simulink model "AccelCtrl_ACC"  (Simulink 7.5)
settings: Solver=ode45  StartTime=0.0  StopTime=inf  RelTol=1e-3
libraries: CarMaker4SL x31, simulink x2
(part 2 of 2)

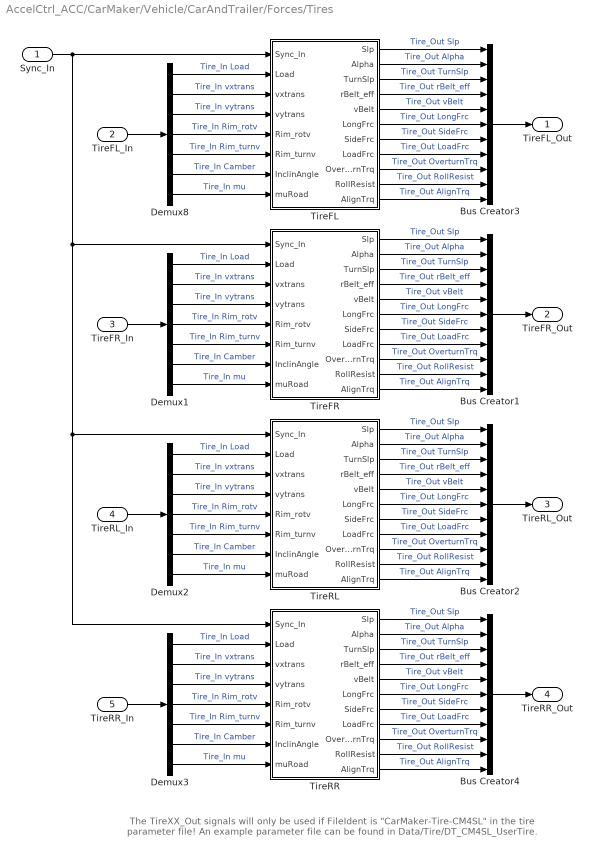
== system AccelCtrl_ACC/CarMaker/Vehicle/CarAndTrailer/Forces/Tires ==
  note: The TireXX_Out signals will only be used if FileIdent is "CarMaker-Tire-CM4SL" in the tire parameter file!
      | An example parameter file can be found in Data/Tire/DT_CM4SL_UserTire.
  Sync_In : Inport  OutDataType=sfix(16)  OutScaling=2^0
  TireFL_In : Inport  Port=2  OutDataType=sfix(16)  OutScaling=2^0
  TireFR_In : Inport  Port=3  OutDataType=sfix(16)  OutScaling=2^0
  TireRL_In : Inport  Port=4  OutDataType=sfix(16)  OutScaling=2^0
  TireRR_In : Inport  Port=5  OutDataType=sfix(16)  OutScaling=2^0
  Bus Creator{1..4} (4 alike) : BusCreator  Inputs=11
  Demux{1..3,8} (4 alike) : Demux  Outputs=7
  TireFL : Subsystem
  TireFR : Subsystem
  TireRL : Subsystem
  TireRR : Subsystem
  TireFL_Out : Outport  OutDataType=sfix(16)  OutScaling=2^0
  TireFR_Out : Outport  Port=2  OutDataType=sfix(16)  OutScaling=2^0
  TireRL_Out : Outport  Port=3  OutDataType=sfix(16)  OutScaling=2^0
  TireRR_Out : Outport  Port=4  OutDataType=sfix(16)  OutScaling=2^0
  wires:
  Sync_In/1 -> TireRR/1(Sync_In), TireRL/1(Sync_In), TireFR/1(Sync_In), TireFL/1(Sync_In)
  Bus Creator4/1 -> TireRR_Out/1
  Bus Creator2/1 -> TireRL_Out/1
  Bus Creator1/1 -> TireFR_Out/1
  Demux3/5 -> TireRR/6(Rim_turnv)  "Tire_In Rim_turnv"
  Demux3/4 -> TireRR/5(Rim_rotv)  "Tire_In Rim_rotv"
  Demux3/1 -> TireRR/2(Load)  "Tire_In Load"
  Demux3/7 -> TireRR/8(muRoad)  "Tire_In mu"
  Demux3/6 -> TireRR/7(InclinAngle)  "Tire_In Camber"
  Demux3/2 -> TireRR/3(vxtrans)  "Tire_In vxtrans"
  Demux3/3 -> TireRR/4(vytrans)  "Tire_In vytrans"
  TireRR/11(AlignTrq) -> Bus Creator4/11  "Tire_Out AlignTrq"
  TireRR/10(RollResist) -> Bus Creator4/10  "Tire_Out RollResist"
  TireRR/9(OverturnTrq) -> Bus Creator4/9  "Tire_Out OverturnTrq"
  TireRR/8(LoadFrc) -> Bus Creator4/8  "Tire_Out LoadFrc"
  TireRR/7(SideFrc) -> Bus Creator4/7  "Tire_Out SideFrc"
  TireRR/6(LongFrc) -> Bus Creator4/6  "Tire_Out LongFrc"
  TireRR/5(vBelt) -> Bus Creator4/5  "Tire_Out vBelt"
  TireRR/4(rBelt_eff) -> Bus Creator4/4  "Tire_Out rBelt_eff"
  TireRR/3(TurnSlp) -> Bus Creator4/3  "Tire_Out TurnSlp"
  TireRR/1(Slp) -> Bus Creator4/1  "Tire_Out Slp"
  TireRR/2(Alpha) -> Bus Creator4/2  "Tire_Out Alpha"
  Demux2/5 -> TireRL/6(Rim_turnv)  "Tire_In Rim_turnv"
  Demux2/4 -> TireRL/5(Rim_rotv)  "Tire_In Rim_rotv"
  Demux2/1 -> TireRL/2(Load)  "Tire_In Load"
  Demux2/7 -> TireRL/8(muRoad)  "Tire_In mu"
  Demux2/6 -> TireRL/7(InclinAngle)  "Tire_In Camber"
  Demux2/2 -> TireRL/3(vxtrans)  "Tire_In vxtrans"
  Demux2/3 -> TireRL/4(vytrans)  "Tire_In vytrans"
  TireRL/11(AlignTrq) -> Bus Creator2/11  "Tire_Out AlignTrq"
  TireRL/10(RollResist) -> Bus Creator2/10  "Tire_Out RollResist"
  TireRL/9(OverturnTrq) -> Bus Creator2/9  "Tire_Out OverturnTrq"
  TireRL/8(LoadFrc) -> Bus Creator2/8  "Tire_Out LoadFrc"
  TireRL/7(SideFrc) -> Bus Creator2/7  "Tire_Out SideFrc"
  TireRL/6(LongFrc) -> Bus Creator2/6  "Tire_Out LongFrc"
  TireRL/5(vBelt) -> Bus Creator2/5  "Tire_Out vBelt"
  TireRL/4(rBelt_eff) -> Bus Creator2/4  "Tire_Out rBelt_eff"
  TireRL/3(TurnSlp) -> Bus Creator2/3  "Tire_Out TurnSlp"
  TireRL/1(Slp) -> Bus Creator2/1  "Tire_Out Slp"
  TireRL/2(Alpha) -> Bus Creator2/2  "Tire_Out Alpha"
  Demux1/5 -> TireFR/6(Rim_turnv)  "Tire_In Rim_turnv"
  Demux1/4 -> TireFR/5(Rim_rotv)  "Tire_In Rim_rotv"
  Demux1/1 -> TireFR/2(Load)  "Tire_In Load"
  Demux1/7 -> TireFR/8(muRoad)  "Tire_In mu"
  Demux1/6 -> TireFR/7(InclinAngle)  "Tire_In Camber"
  Demux1/2 -> TireFR/3(vxtrans)  "Tire_In vxtrans"
  Demux1/3 -> TireFR/4(vytrans)  "Tire_In vytrans"
  TireFR/11(AlignTrq) -> Bus Creator1/11  "Tire_Out AlignTrq"
  TireFR/10(RollResist) -> Bus Creator1/10  "Tire_Out RollResist"
  TireFR/9(OverturnTrq) -> Bus Creator1/9  "Tire_Out OverturnTrq"
  TireFR/8(LoadFrc) -> Bus Creator1/8  "Tire_Out LoadFrc"
  TireFR/7(SideFrc) -> Bus Creator1/7  "Tire_Out SideFrc"
  TireFR/6(LongFrc) -> Bus Creator1/6  "Tire_Out LongFrc"
  TireFR/5(vBelt) -> Bus Creator1/5  "Tire_Out vBelt"
  TireFR/4(rBelt_eff) -> Bus Creator1/4  "Tire_Out rBelt_eff"
  TireFR/3(TurnSlp) -> Bus Creator1/3  "Tire_Out TurnSlp"
  TireFR/1(Slp) -> Bus Creator1/1  "Tire_Out Slp"
  TireFR/2(Alpha) -> Bus Creator1/2  "Tire_Out Alpha"
  Demux8/5 -> TireFL/6(Rim_turnv)  "Tire_In Rim_turnv"
  Demux8/4 -> TireFL/5(Rim_rotv)  "Tire_In Rim_rotv"
  TireFL_In/1 -> Demux8/1
  Demux8/1 -> TireFL/2(Load)  "Tire_In Load"
  Demux8/7 -> TireFL/8(muRoad)  "Tire_In mu"
  Demux8/6 -> TireFL/7(InclinAngle)  "Tire_In Camber"
  Demux8/2 -> TireFL/3(vxtrans)  "Tire_In vxtrans"
  Demux8/3 -> TireFL/4(vytrans)  "Tire_In vytrans"
  TireFL/11(AlignTrq) -> Bus Creator3/11  "Tire_Out AlignTrq"
  TireFL/10(RollResist) -> Bus Creator3/10  "Tire_Out RollResist"
  TireFL/9(OverturnTrq) -> Bus Creator3/9  "Tire_Out OverturnTrq"
  TireFL/8(LoadFrc) -> Bus Creator3/8  "Tire_Out LoadFrc"
  TireFL/7(SideFrc) -> Bus Creator3/7  "Tire_Out SideFrc"
  TireFL/6(LongFrc) -> Bus Creator3/6  "Tire_Out LongFrc"
  TireFL/5(vBelt) -> Bus Creator3/5  "Tire_Out vBelt"
  TireFL/4(rBelt_eff) -> Bus Creator3/4  "Tire_Out rBelt_eff"
  TireFL/3(TurnSlp) -> Bus Creator3/3  "Tire_Out TurnSlp"
  TireFL/1(Slp) -> Bus Creator3/1  "Tire_Out Slp"
  TireFL/2(Alpha) -> Bus Creator3/2  "Tire_Out Alpha"
  Bus Creator3/1 -> TireFL_Out/1
  TireFR_In/1 -> Demux1/1
  TireRL_In/1 -> Demux2/1
  TireRR_In/1 -> Demux3/1

== system AccelCtrl_ACC/CarMaker/Vehicle/CarAndTrailer/Forces/Vehicle Forces ==
  Sync_In : Inport  OutDataType=sfix(16)  OutScaling=2^0
  Bus Creator1 : BusCreator  Inputs=12
  Bus Creator5 : BusCreator  Inputs=13
  Bus Creator8 : BusCreator  Inputs=16
  Demux : Demux  Outputs=16
  Demux1 : Demux  Outputs=12
  Demux5 : Demux  Outputs=13
  Forces : S-Function  FunctionName=CM_Sfun  Parameters='Forces'  EnableBusSupport=off
  Sync_Out : Outport  OutDataType=sfix(16)  OutScaling=2^0
  Car.Virtual : Outport  Port=2  OutDataType=sfix(16)  OutScaling=2^0
  Car.Aero : Outport  Port=3  OutDataType=sfix(16)  OutScaling=2^0
  Car.Load : Outport  Port=4  OutDataType=sfix(16)  OutScaling=2^0
  wires:
  Demux5/7 -> Bus Creator5/7  "car Aero vRes_1 z"
  Demux5/6 -> Bus Creator5/6  "car Aero vRes_1 y"
  Demux5/5 -> Bus Creator5/5  "car Aero vRes_1 x"
  Demux5/4 -> Bus Creator5/4  "Vehicle Wind_vel_0 z"
  Demux5/3 -> Bus Creator5/3  "Vehicle Wind_vel_0 y"
  Demux5/2 -> Bus Creator5/2  "Vehicle Wind_vel_0 x"
  Demux5/1 -> Bus Creator5/1  "Vehicle sRoadAero"
  Demux5/8 -> Bus Creator5/8  "car Aero Frc_1 x"
  Demux5/9 -> Bus Creator5/9  "car Aero Frc_1 y"
  Demux5/10 -> Bus Creator5/10  "car Aero Frc_1 z"
  Demux5/13 -> Bus Creator5/13  "car Aero Trq_1 z"
  Demux5/12 -> Bus Creator5/12  "car Aero Trq_1 y"
  Demux5/11 -> Bus Creator5/11  "car Aero Trq_1 x"
  Forces/4 -> Demux/1
  Demux/12 -> Bus Creator8/12  "Car Load_2 tz"
  Demux/11 -> Bus Creator8/11  "Car Load_2 ty"
  Demux/10 -> Bus Creator8/10  "Car Load_2 tx"
  Demux/9 -> Bus Creator8/9  "Car Load_2 mass"
  Demux/8 -> Bus Creator8/8  "Car Load_1 tz"
  Demux/7 -> Bus Creator8/7  "Car Load_1 ty"
  Demux/6 -> Bus Creator8/6  "Car Load_1 tx"
  Demux/5 -> Bus Creator8/5  "Car Load_1 mass"
  Demux/4 -> Bus Creator8/4  "Car Load_0 tz"
  Demux/3 -> Bus Creator8/3  "Car Load_0 ty"
  Demux/2 -> Bus Creator8/2  "Car Load_0 tx"
  Demux/1 -> Bus Creator8/1  "Car Load_0 mass"
  Bus Creator8/1 -> Car.Load/1
  Bus Creator1/1 -> Car.Virtual/1
  Forces/2 -> Demux1/1
  Forces/3 -> Demux5/1
  Demux1/3 -> Bus Creator1/3  "Car Virtual Frc_1 z"
  Demux1/2 -> Bus Creator1/2  "Car Virtual Frc_1 y"
  Demux1/1 -> Bus Creator1/1  "Car Virtual Frc_1 x"
  Bus Creator5/1 -> Car.Aero/1
  Forces/1 -> Sync_Out/1
  Sync_In/1 -> Forces/1
  Demux1/4 -> Bus Creator1/4  "Car Virtual Frc_0 x"
  Demux1/5 -> Bus Creator1/5  "Car Virtual Frc_0 y"
  Demux1/6 -> Bus Creator1/6  "Car Virtual Frc_0 z"
  Demux1/7 -> Bus Creator1/7  "Car Virtual Trq_1 x"
  Demux1/8 -> Bus Creator1/8  "Car Virtual Trq_1 y"
  Demux1/9 -> Bus Creator1/9  "Car Virtual Trq_1 z"
  Demux1/10 -> Bus Creator1/10  "Car Virtual Trq_0 x"
  Demux1/11 -> Bus Creator1/11  "Car Virtual Trq_0 y"
  Demux1/12 -> Bus Creator1/12  "Car Virtual Trq_0 z"
  Demux/13 -> Bus Creator8/13  "Car Load_3 mass"
  Demux/14 -> Bus Creator8/14  "Car Load_3 tx"
  Demux/15 -> Bus Creator8/15  "Car Load_3 ty"
  Demux/16 -> Bus Creator8/16  "Car Load_3 tz"

== system AccelCtrl_ACC/CarMaker/Vehicle/CarAndTrailer/Trailer/CreateBus Car.Hitch.FrcTrq ==
  In1 : Inport  OutDataType=sfix(16)  OutScaling=2^0
  Bus Creator7 : BusCreator  Inputs=6
  Demux7 : Demux  Outputs=6
  Car.Hitch.FrcTrq : Outport  OutDataType=sfix(16)  OutScaling=2^0
  wires:
  Demux7/1 -> Bus Creator7/1  "Car Hitch Frc2Car x"
  Demux7/2 -> Bus Creator7/2  "Car Hitch Frc2Car y"
  Demux7/3 -> Bus Creator7/3  "Car Hitch Frc2Car z"
  Demux7/4 -> Bus Creator7/4  "Car Hitch Trq2Car x"
  Demux7/5 -> Bus Creator7/5  "Car Hitch Trq2Car y"
  Demux7/6 -> Bus Creator7/6  "Car Hitch Trq2Car z"
  Bus Creator7/1 -> Car.Hitch.FrcTrq/1
  In1/1 -> Demux7/1

== system AccelCtrl_ACC/CarMaker/Vehicle/CarAndTrailer/Trailer/CreateBus Vhcl.Motion ==
  In1 : Inport  OutDataType=sfix(16)  OutScaling=2^0
  Demux1 : Demux  Outputs=16
  Mux1 : Mux  Inputs=16
  Out1 : Outport  OutDataType=sfix(16)  OutScaling=2^0
  wires:
  Mux1/1 -> Out1/1
  In1/1 -> Demux1/1
  Demux1/16 -> Mux1/16  "Vhcl YawAcc"
  Demux1/15 -> Mux1/15  "Vhcl YawRate"
  Demux1/14 -> Mux1/14  "Vhcl Yaw"
  Demux1/13 -> Mux1/13  "Vhcl PitchAcc"
  Demux1/12 -> Mux1/12  "Vhcl PitchVel"
  Demux1/11 -> Mux1/11  "Vhcl Pitch"
  Demux1/10 -> Mux1/10  "Vhcl RollAcc"
  Demux1/9 -> Mux1/9  "Vhcl RollVel"
  Demux1/8 -> Mux1/8  "Vhcl Roll"
  Demux1/7 -> Mux1/7  "Vhcl Hitch_Pos z"
  Demux1/6 -> Mux1/6  "Vhcl Hitch_Pos y"
  Demux1/5 -> Mux1/5  "Vhcl Hitch_Pos x"
  Demux1/4 -> Mux1/4  "Vhcl sRoadAero"
  Demux1/3 -> Mux1/3  "Vhcl sRoad"
  Demux1/2 -> Mux1/2  "Vhcl Distance"
  Demux1/1 -> Mux1/1  "Vhcl v"

== system AccelCtrl_ACC/CarMaker/Vehicle/CarAndTrailer/Trailer/CreateBus Vhcl.PoI ==
  In1 : Inport  OutDataType=sfix(16)  OutScaling=2^0
  Bus Creator3 : BusCreator  Inputs=18
  Demux3 : Demux  Outputs=18
  Out1 : Outport  OutDataType=sfix(16)  OutScaling=2^0
  wires:
  Demux3/1 -> Bus Creator3/1  "Vhcl PoI_Pos x"
  Bus Creator3/1 -> Out1/1
  In1/1 -> Demux3/1
  Demux3/2 -> Bus Creator3/2  "Vhcl PoI_Pos y"
  Demux3/3 -> Bus Creator3/3  "Vhcl PoI_Pos z"
  Demux3/4 -> Bus Creator3/4  "Vhcl PoI_Vel x"
  Demux3/5 -> Bus Creator3/5  "Vhcl PoI_Vel y"
  Demux3/6 -> Bus Creator3/6  "Vhcl PoI_Vel z"
  Demux3/7 -> Bus Creator3/7  "Vhcl PoI_Acc x"
  Demux3/8 -> Bus Creator3/8  "Vhcl PoI_Acc y"
  Demux3/9 -> Bus Creator3/9  "Vhcl PoI_Acc z"
  Demux3/10 -> Bus Creator3/10  "Vhcl PoI_Vel_1 x"
  Demux3/11 -> Bus Creator3/11  "Vhcl PoI_Vel_1 y"
  Demux3/12 -> Bus Creator3/12  "Vhcl PoI_Vel_1 z"
  Demux3/13 -> Bus Creator3/13  "Vhcl PoI_Acc_1 x"
  Demux3/14 -> Bus Creator3/14  "Vhcl PoI_Acc_1 y"
  Demux3/15 -> Bus Creator3/15  "Vhcl PoI_Acc_1 z"
  Demux3/16 -> Bus Creator3/16  "Vhcl PoI_GCS Long"
  Demux3/17 -> Bus Creator3/17  "Vhcl PoI_GCS Lat"
  Demux3/18 -> Bus Creator3/18  "Vhcl PoI_GCS Elev"

== system AccelCtrl_ACC/CarMaker/Vehicle/CarAndTrailer/Trailer/CreateBus Vhcl.Steering ==
  In1 : Inport  OutDataType=sfix(16)  OutScaling=2^0
  Bus Creator3 : BusCreator
  Demux : Demux
  Out1 : Outport  OutDataType=sfix(16)  OutScaling=2^0
  wires:
  In1/1 -> Demux/1
  Demux/4 -> Bus Creator3/4  "Vhcl Steering Trq"
  Demux/2 -> Bus Creator3/2  "Vhcl Steering AngVel"
  Demux/3 -> Bus Creator3/3  "Vhcl Steering AngAcc"
  Demux/1 -> Bus Creator3/1  "Vhcl Steering Ang"
  Bus Creator3/1 -> Out1/1

== system AccelCtrl_ACC/CarMaker/Vehicle/CarAndTrailer/Trailer/CreateBus Vhcl.Wheel.FL ==
  In1 : Inport  OutDataType=sfix(16)  OutScaling=2^0
  Bus Creator3 : BusCreator  Inputs=14
  Demux3 : Demux  Outputs=14
  Out1 : Outport  OutDataType=sfix(16)  OutScaling=2^0
  wires:
  Demux3/1 -> Bus Creator3/1  "Vhcl Wheel FL t x"
  Bus Creator3/1 -> Out1/1
  In1/1 -> Demux3/1
  Demux3/2 -> Bus Creator3/2  "Vhcl Wheel FL t y"
  Demux3/3 -> Bus Creator3/3  "Vhcl Wheel FL t z"
  Demux3/4 -> Bus Creator3/4  "Vhcl Wheel FL r_zxy x"
  Demux3/5 -> Bus Creator3/5  "Vhcl Wheel FL r_zxy y"
  Demux3/6 -> Bus Creator3/6  "Vhcl Wheel FL r_zxy z"
  Demux3/7 -> Bus Creator3/7  "Vhcl Wheel FL Fx"
  Demux3/8 -> Bus Creator3/8  "Vhcl Wheel FL Fy"
  Demux3/9 -> Bus Creator3/9  "Vhcl Wheel FL Fz"
  Demux3/10 -> Bus Creator3/10  "Vhcl Wheel FL vBelt"
  Demux3/11 -> Bus Creator3/11  "Vhcl Wheel FL LongSlip"
  Demux3/12 -> Bus Creator3/12  "Vhcl Wheel FL SideSlip"
  Demux3/13 -> Bus Creator3/13  "Vhcl Wheel FL Trq_T2W"
  Demux3/14 -> Bus Creator3/14  "Vhcl Wheel FL Trq_WhlBearing"

== system AccelCtrl_ACC/CarMaker/Vehicle/CarAndTrailer/Trailer/CreateBus Vhcl.Wheel.FR ==
  In1 : Inport  OutDataType=sfix(16)  OutScaling=2^0
  Bus Creator3 : BusCreator  Inputs=14
  Demux3 : Demux  Outputs=14
  Out1 : Outport  OutDataType=sfix(16)  OutScaling=2^0
  wires:
  Demux3/1 -> Bus Creator3/1  "Vhcl Wheel FR t x"
  Bus Creator3/1 -> Out1/1
  In1/1 -> Demux3/1
  Demux3/2 -> Bus Creator3/2  "Vhcl Wheel FR t y"
  Demux3/3 -> Bus Creator3/3  "Vhcl Wheel FR t z"
  Demux3/4 -> Bus Creator3/4  "Vhcl Wheel FR r_zxy x"
  Demux3/5 -> Bus Creator3/5  "Vhcl Wheel FR r_zxy y"
  Demux3/6 -> Bus Creator3/6  "Vhcl Wheel FR r_zxy z"
  Demux3/7 -> Bus Creator3/7  "Vhcl Wheel FR Fx"
  Demux3/8 -> Bus Creator3/8  "Vhcl Wheel FR Fy"
  Demux3/9 -> Bus Creator3/9  "Vhcl Wheel FR Fz"
  Demux3/10 -> Bus Creator3/10  "Vhcl Wheel FR vBelt"
  Demux3/11 -> Bus Creator3/11  "Vhcl Wheel FR LongSlip"
  Demux3/12 -> Bus Creator3/12  "Vhcl Wheel FR SideSlip"
  Demux3/13 -> Bus Creator3/13  "Vhcl Wheel FR Trq_T2W"
  Demux3/14 -> Bus Creator3/14  "Vhcl Wheel FR Trq_WhlBearing"

== system AccelCtrl_ACC/CarMaker/Vehicle/CarAndTrailer/Trailer/CreateBus Vhcl.Wheel.RL ==
  In1 : Inport  OutDataType=sfix(16)  OutScaling=2^0
  Bus Creator3 : BusCreator  Inputs=14
  Demux3 : Demux  Outputs=14
  Out1 : Outport  OutDataType=sfix(16)  OutScaling=2^0
  wires:
  Demux3/1 -> Bus Creator3/1  "Vhcl Wheel RL t x"
  Bus Creator3/1 -> Out1/1
  In1/1 -> Demux3/1
  Demux3/2 -> Bus Creator3/2  "Vhcl Wheel RL t y"
  Demux3/3 -> Bus Creator3/3  "Vhcl Wheel RL t z"
  Demux3/4 -> Bus Creator3/4  "Vhcl Wheel RL r_zxy x"
  Demux3/5 -> Bus Creator3/5  "Vhcl Wheel RL r_zxy y"
  Demux3/6 -> Bus Creator3/6  "Vhcl Wheel RL r_zxy z"
  Demux3/7 -> Bus Creator3/7  "Vhcl Wheel RL Fx"
  Demux3/8 -> Bus Creator3/8  "Vhcl Wheel RL Fy"
  Demux3/9 -> Bus Creator3/9  "Vhcl Wheel RL Fz"
  Demux3/10 -> Bus Creator3/10  "Vhcl Wheel RL vBelt"
  Demux3/11 -> Bus Creator3/11  "Vhcl Wheel RL LongSlip"
  Demux3/12 -> Bus Creator3/12  "Vhcl Wheel RL SideSlip"
  Demux3/13 -> Bus Creator3/13  "Vhcl Wheel RL Trq_T2W"
  Demux3/14 -> Bus Creator3/14  "Vhcl Wheel RL Trq_WhlBearing"

== system AccelCtrl_ACC/CarMaker/Vehicle/CarAndTrailer/Trailer/CreateBus Vhcl.Wheel.RR ==
  In1 : Inport  OutDataType=sfix(16)  OutScaling=2^0
  Bus Creator3 : BusCreator  Inputs=14
  Demux3 : Demux  Outputs=14
  Out1 : Outport  OutDataType=sfix(16)  OutScaling=2^0
  wires:
  Demux3/1 -> Bus Creator3/1  "Vhcl Wheel RR t x"
  Bus Creator3/1 -> Out1/1
  In1/1 -> Demux3/1
  Demux3/2 -> Bus Creator3/2  "Vhcl Wheel RR t y"
  Demux3/3 -> Bus Creator3/3  "Vhcl Wheel RR t z"
  Demux3/4 -> Bus Creator3/4  "Vhcl Wheel RR r_zxy x"
  Demux3/5 -> Bus Creator3/5  "Vhcl Wheel RR r_zxy y"
  Demux3/6 -> Bus Creator3/6  "Vhcl Wheel RR r_zxy z"
  Demux3/7 -> Bus Creator3/7  "Vhcl Wheel RR Fx"
  Demux3/8 -> Bus Creator3/8  "Vhcl Wheel RR Fy"
  Demux3/9 -> Bus Creator3/9  "Vhcl Wheel RR Fz"
  Demux3/10 -> Bus Creator3/10  "Vhcl Wheel RR vBelt"
  Demux3/11 -> Bus Creator3/11  "Vhcl Wheel RR LongSlip"
  Demux3/12 -> Bus Creator3/12  "Vhcl Wheel RR SideSlip"
  Demux3/13 -> Bus Creator3/13  "Vhcl Wheel RR Trq_T2W"
  Demux3/14 -> Bus Creator3/14  "Vhcl Wheel RR Trq_WhlBearing"

== system AccelCtrl_ACC/CarMaker/VehicleControl/AccelCtrl/ACC ECU/ACC Control ==
  ACC enabled : Inport  OutDataType=sfix(16)  OutScaling=2^0
  Target Dtct : Inport  Port=2  OutDataType=sfix(16)  OutScaling=2^0
  Target.ds : Inport  Port=3  OutDataType=sfix(16)  OutScaling=2^0
  Target.dv : Inport  Port=4  OutDataType=sfix(16)  OutScaling=2^0
  Desired time gap : Inport  Port=5  OutDataType=sfix(16)  OutScaling=2^0
  Desired speed : Inport  Port=6  OutDataType=sfix(16)  OutScaling=2^0
  Desired Distance Calculation with time gap : Subsystem  TreatAsAtomicUnit=on
  Distance Control Algorithm : Subsystem  TreatAsAtomicUnit=on
  Logical Operator : Logic  AllPortsSameDT=off
  Speed Control Algorithm : Subsystem  TreatAsAtomicUnit=on
  Target detected : simulink/Logic and Bit Operations/Compare To Zero  SystemSampleTime=-1  relop=>  LogicOutDataTypeMode=uint8  ZeroCross=off
  Zero Ax : Constant  Value=0  OutDataType=sfix(16)  OutScaling=2^0
  desired ax : Switch  Threshold=1  SaturateOnIntegerOverflow=on
  desired or zero : Switch  Threshold=1  SaturateOnIntegerOverflow=on
  Desired Ax : Outport  OutDataType=sfix(16)  OutScaling=2^0
  wires:
  Zero Ax/1 -> desired or zero/3
  desired ax/1 -> desired or zero/1
  desired or zero/1 -> Desired Ax/1
  Logical Operator/1 -> Desired Distance Calculation with time gap/Enable
  ACC enabled/1 -> desired or zero/2, Logical Operator/1
  Speed Control Algorithm/1(ax speed control) -> Distance Control Algorithm/4(ax speed control), desired ax/3
  Desired speed/1 -> Speed Control Algorithm/1(desire speed[m/s])
  Desired time gap/1 -> Desired Distance Calculation with time gap/2(desired time gap)
  Desired Distance Calculation with time gap/1(desired distance) -> Distance Control Algorithm/3(desired distance[m])
  Target detected/1 -> Logical Operator/2, desired ax/2
  Distance Control Algorithm/1("  limited ax") -> desired ax/1
  Target Dtct/1 -> Target detected/1
  Target.ds/1 -> Distance Control Algorithm/1(Target.ds[m])
  Target.dv/1 -> Desired Distance Calculation with time gap/1(Target.dv), Distance Control Algorithm/2(Target.dv[m/s])

== system AccelCtrl_ACC/CarMaker/VehicleControl/AccelCtrl/ACC ECU/ACC User Input ==
  ACC Active ACC/Actual Speed : Switch  Threshold=1  SaturateOnIntegerOverflow=on
  Constant : Constant  OutDataType=sfix(16)  OutScaling=2^0
  Init Desired time gap quantity : Subsystem  TreatAsAtomicUnit=on
  Is ACC enabled : CarMaker4SL/Read CM Dict  xname=AccelCtrl.ACC.IsActive  xsync=off
  Memory : Memory
  Read Car.v[m/s] : CarMaker4SL/Read CM Dict  xname=Car.v  xsync=off
  Read User desired speed : CarMaker4SL/Read CM Dict  xname=AccelCtrl.ACC.DesiredSpd  xsync=off
  Read User desired time gap : CarMaker4SL/Read CM Dict  xname=AccelCtrl.ACC.DesiredTGap  xsync=off
  Read init desired time gap from Inf : CarMaker4SL/Read CM Parameter  xfile=Vehicle  xkey=AccelCtrl.ACC.DesrTGap  xnout=1  xdefaults=1.8  xmuxed=off
  Write desired speed : CarMaker4SL/Write CM Dict  xname=AccelCtrl.ACC.DesiredSpd  xsync=off
  ACC enabled : Outport  OutDataType=sfix(16)  OutScaling=2^0
  Desired time gap[s] : Outport  Port=2  OutDataType=sfix(16)  OutScaling=2^0
  Desired speed[m/s] : Outport  Port=3  OutDataType=sfix(16)  OutScaling=2^0
  wires:
  Read init desired time gap from Inf/1 -> Init Desired time gap quantity/1("Init desired time gap ")
  Memory/1 -> Init Desired time gap quantity/Trigger
  Constant/1 -> Memory/1
  Read User desired time gap/1 -> Desired time gap[s]/1
  ACC Active ACC/Actual Speed/1 -> Write desired speed/1, Desired speed[m/s]/1
  Read Car.v[m/s]/1 -> ACC Active ACC/Actual Speed/3
  Read User desired speed/1 -> ACC Active ACC/Actual Speed/1
  Is ACC enabled/1 -> ACC Active ACC/Actual Speed/2, ACC enabled/1

== system AccelCtrl_ACC/CarMaker/VehicleControl/AccelCtrl/AccelCtrl/PI-Controller ==
  delta_ax : Inport  OutDataType=sfix(16)  OutScaling=2^0
  DM_Gas : Inport  Port=2  OutDataType=sfix(16)  OutScaling=2^0
  AxCtrl On : Inport  Port=3  OutDataType=sfix(16)  OutScaling=2^0
  Add : Sum  OutDataType=sfix(16)  OutScaling=2^-10  SaturateOnIntegerOverflow=on  OutDataTypeStr=Inherit: Same as first input
  Integrator : Subsystem
  Read init i_gain from Inf : CarMaker4SL/Read CM Parameter  xfile=Vehicle  xkey=AccelCtrl.i_gain  xnout=1  xdefaults=0.001  xmuxed=off
  Read init p_gain from Inf : CarMaker4SL/Read CM Parameter  xfile=Vehicle  xkey=AccelCtrl.p_gain  xnout=1  xdefaults=0.001  xmuxed=off
  Saturation : Saturate  UpperLimit=1  LowerLimit=-1
  i_gain : Product  OutDataType=sfix(16)  OutScaling=2^0  SaturateOnIntegerOverflow=on  OutDataTypeStr=Inherit: Same as first input
  p_gain : Product  OutDataType=sfix(16)  OutScaling=2^0  SaturateOnIntegerOverflow=on  OutDataTypeStr=Inherit: Same as first input
  Gas or Brake : Outport  OutDataType=sfix(16)  OutScaling=2^0
  wires:
  Read init i_gain from Inf/1 -> i_gain/2
  Read init p_gain from Inf/1 -> p_gain/1
  Integrator/1("I-part tot ") -> Add/2
  DM_Gas/1 -> Integrator/3(Init I-part)
  AxCtrl On/1 -> Integrator/2(AxCtrl On)
  i_gain/1 -> Integrator/1(I-Part)
  delta_ax/1 -> i_gain/1, p_gain/2
  p_gain/1 -> Add/1
  Add/1 -> Saturation/1
  Saturation/1 -> Gas or Brake/1

== system AccelCtrl_ACC/CarMaker/VehicleControl/AccelCtrl/AccelCtrl/controlled process variable  ==
  desired ax : Inport  OutDataType=sfix(16)  OutScaling=2^0
  Read Car.ax : CarMaker4SL/Read CM Dict  xname=Car.ax  xsync=off
  Subtract : Sum  Inputs=+-  OutDataType=sfix(16)  OutScaling=2^-10  SaturateOnIntegerOverflow=on
  delta ax : Outport  OutDataType=sfix(16)  OutScaling=2^0
  wires:
  Subtract/1 -> delta ax/1
  Read Car.ax/1 -> Subtract/2
  desired ax/1 -> Subtract/1

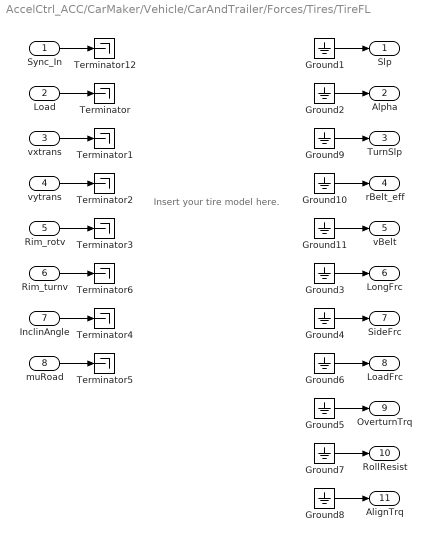
== system AccelCtrl_ACC/CarMaker/Vehicle/CarAndTrailer/Forces/Tires/TireFL ==
  note: Insert your tire model here.
  Sync_In : Inport  OutDataType=sfix(16)  OutScaling=2^0
  Load : Inport  Port=2  OutDataType=sfix(16)  OutScaling=2^0
  vxtrans : Inport  Port=3  OutDataType=sfix(16)  OutScaling=2^0
  vytrans : Inport  Port=4  OutDataType=sfix(16)  OutScaling=2^0
  Rim_rotv : Inport  Port=5  OutDataType=sfix(16)  OutScaling=2^0
  Rim_turnv : Inport  Port=6  OutDataType=sfix(16)  OutScaling=2^0
  InclinAngle : Inport  Port=7  OutDataType=sfix(16)  OutScaling=2^0
  muRoad : Inport  Port=8  OutDataType=sfix(16)  OutScaling=2^0
  Ground{1..11} (11 alike) : Ground
  Terminator{,1..6,12} (8 alike) : Terminator
  Slp : Outport  OutDataType=sfix(16)  OutScaling=2^0
  Alpha : Outport  Port=2  OutDataType=sfix(16)  OutScaling=2^0
  TurnSlp : Outport  Port=3  OutDataType=sfix(16)  OutScaling=2^0
  rBelt_eff : Outport  Port=4  OutDataType=sfix(16)  OutScaling=2^0
  vBelt : Outport  Port=5  OutDataType=sfix(16)  OutScaling=2^0
  LongFrc : Outport  Port=6  OutDataType=sfix(16)  OutScaling=2^0
  SideFrc : Outport  Port=7  OutDataType=sfix(16)  OutScaling=2^0
  LoadFrc : Outport  Port=8  OutDataType=sfix(16)  OutScaling=2^0
  OverturnTrq : Outport  Port=9  OutDataType=sfix(16)  OutScaling=2^0
  RollResist : Outport  Port=10  OutDataType=sfix(16)  OutScaling=2^0
  AlignTrq : Outport  Port=11  OutDataType=sfix(16)  OutScaling=2^0
  wires:
  Ground11/1 -> vBelt/1
  Ground10/1 -> rBelt_eff/1
  Ground9/1 -> TurnSlp/1
  Rim_turnv/1 -> Terminator6/1
  Sync_In/1 -> Terminator12/1
  Ground2/1 -> Alpha/1
  Ground3/1 -> LongFrc/1
  Ground4/1 -> SideFrc/1
  Ground5/1 -> OverturnTrq/1
  vxtrans/1 -> Terminator1/1
  vytrans/1 -> Terminator2/1
  Rim_rotv/1 -> Terminator3/1
  InclinAngle/1 -> Terminator4/1
  muRoad/1 -> Terminator5/1
  Load/1 -> Terminator/1
  Ground1/1 -> Slp/1
  Ground6/1 -> LoadFrc/1
  Ground7/1 -> RollResist/1
  Ground8/1 -> AlignTrq/1

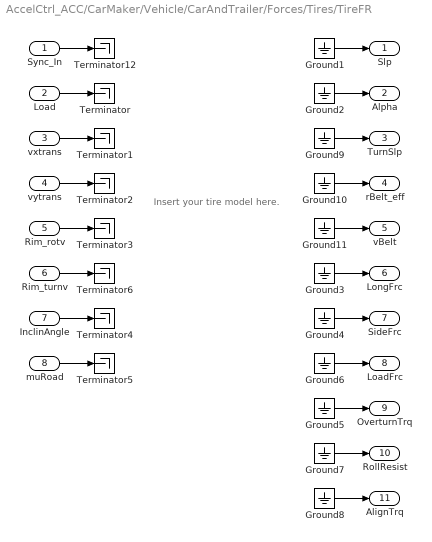
== system AccelCtrl_ACC/CarMaker/Vehicle/CarAndTrailer/Forces/Tires/TireFR ==
  note: Insert your tire model here.
  Sync_In : Inport  OutDataType=sfix(16)  OutScaling=2^0
  Load : Inport  Port=2  OutDataType=sfix(16)  OutScaling=2^0
  vxtrans : Inport  Port=3  OutDataType=sfix(16)  OutScaling=2^0
  vytrans : Inport  Port=4  OutDataType=sfix(16)  OutScaling=2^0
  Rim_rotv : Inport  Port=5  OutDataType=sfix(16)  OutScaling=2^0
  Rim_turnv : Inport  Port=6  OutDataType=sfix(16)  OutScaling=2^0
  InclinAngle : Inport  Port=7  OutDataType=sfix(16)  OutScaling=2^0
  muRoad : Inport  Port=8  OutDataType=sfix(16)  OutScaling=2^0
  Ground{1..11} (11 alike) : Ground
  Terminator{,1..6,12} (8 alike) : Terminator
  Slp : Outport  OutDataType=sfix(16)  OutScaling=2^0
  Alpha : Outport  Port=2  OutDataType=sfix(16)  OutScaling=2^0
  TurnSlp : Outport  Port=3  OutDataType=sfix(16)  OutScaling=2^0
  rBelt_eff : Outport  Port=4  OutDataType=sfix(16)  OutScaling=2^0
  vBelt : Outport  Port=5  OutDataType=sfix(16)  OutScaling=2^0
  LongFrc : Outport  Port=6  OutDataType=sfix(16)  OutScaling=2^0
  SideFrc : Outport  Port=7  OutDataType=sfix(16)  OutScaling=2^0
  LoadFrc : Outport  Port=8  OutDataType=sfix(16)  OutScaling=2^0
  OverturnTrq : Outport  Port=9  OutDataType=sfix(16)  OutScaling=2^0
  RollResist : Outport  Port=10  OutDataType=sfix(16)  OutScaling=2^0
  AlignTrq : Outport  Port=11  OutDataType=sfix(16)  OutScaling=2^0
  wires:
  Ground11/1 -> vBelt/1
  Ground10/1 -> rBelt_eff/1
  Ground9/1 -> TurnSlp/1
  Rim_turnv/1 -> Terminator6/1
  Sync_In/1 -> Terminator12/1
  Ground2/1 -> Alpha/1
  Ground3/1 -> LongFrc/1
  Ground4/1 -> SideFrc/1
  Ground5/1 -> OverturnTrq/1
  vxtrans/1 -> Terminator1/1
  vytrans/1 -> Terminator2/1
  Rim_rotv/1 -> Terminator3/1
  InclinAngle/1 -> Terminator4/1
  muRoad/1 -> Terminator5/1
  Load/1 -> Terminator/1
  Ground1/1 -> Slp/1
  Ground6/1 -> LoadFrc/1
  Ground7/1 -> RollResist/1
  Ground8/1 -> AlignTrq/1

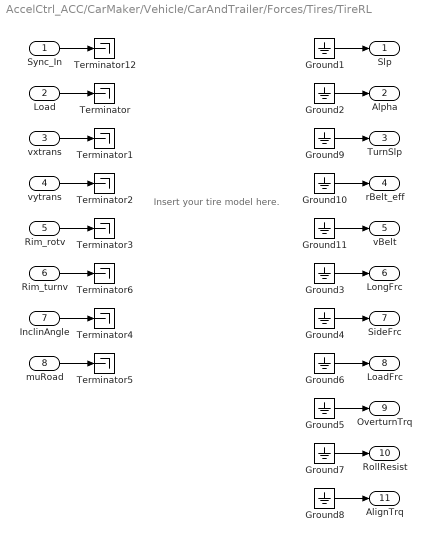
== system AccelCtrl_ACC/CarMaker/Vehicle/CarAndTrailer/Forces/Tires/TireRL ==
  note: Insert your tire model here.
  Sync_In : Inport  OutDataType=sfix(16)  OutScaling=2^0
  Load : Inport  Port=2  OutDataType=sfix(16)  OutScaling=2^0
  vxtrans : Inport  Port=3  OutDataType=sfix(16)  OutScaling=2^0
  vytrans : Inport  Port=4  OutDataType=sfix(16)  OutScaling=2^0
  Rim_rotv : Inport  Port=5  OutDataType=sfix(16)  OutScaling=2^0
  Rim_turnv : Inport  Port=6  OutDataType=sfix(16)  OutScaling=2^0
  InclinAngle : Inport  Port=7  OutDataType=sfix(16)  OutScaling=2^0
  muRoad : Inport  Port=8  OutDataType=sfix(16)  OutScaling=2^0
  Ground{1..11} (11 alike) : Ground
  Terminator{,1..6,12} (8 alike) : Terminator
  Slp : Outport  OutDataType=sfix(16)  OutScaling=2^0
  Alpha : Outport  Port=2  OutDataType=sfix(16)  OutScaling=2^0
  TurnSlp : Outport  Port=3  OutDataType=sfix(16)  OutScaling=2^0
  rBelt_eff : Outport  Port=4  OutDataType=sfix(16)  OutScaling=2^0
  vBelt : Outport  Port=5  OutDataType=sfix(16)  OutScaling=2^0
  LongFrc : Outport  Port=6  OutDataType=sfix(16)  OutScaling=2^0
  SideFrc : Outport  Port=7  OutDataType=sfix(16)  OutScaling=2^0
  LoadFrc : Outport  Port=8  OutDataType=sfix(16)  OutScaling=2^0
  OverturnTrq : Outport  Port=9  OutDataType=sfix(16)  OutScaling=2^0
  RollResist : Outport  Port=10  OutDataType=sfix(16)  OutScaling=2^0
  AlignTrq : Outport  Port=11  OutDataType=sfix(16)  OutScaling=2^0
  wires:
  Ground11/1 -> vBelt/1
  Ground10/1 -> rBelt_eff/1
  Ground9/1 -> TurnSlp/1
  Rim_turnv/1 -> Terminator6/1
  Sync_In/1 -> Terminator12/1
  Ground2/1 -> Alpha/1
  Ground3/1 -> LongFrc/1
  Ground4/1 -> SideFrc/1
  Ground5/1 -> OverturnTrq/1
  vxtrans/1 -> Terminator1/1
  vytrans/1 -> Terminator2/1
  Rim_rotv/1 -> Terminator3/1
  InclinAngle/1 -> Terminator4/1
  muRoad/1 -> Terminator5/1
  Load/1 -> Terminator/1
  Ground1/1 -> Slp/1
  Ground6/1 -> LoadFrc/1
  Ground7/1 -> RollResist/1
  Ground8/1 -> AlignTrq/1

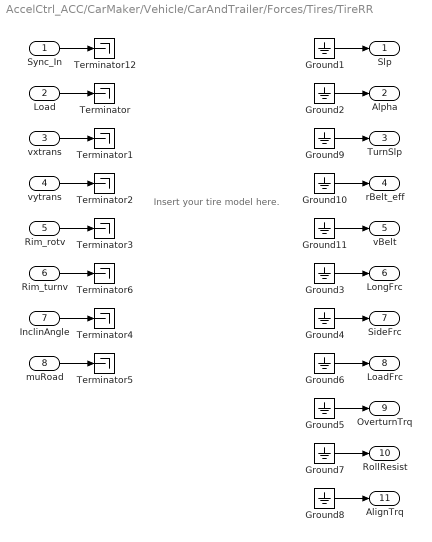
== system AccelCtrl_ACC/CarMaker/Vehicle/CarAndTrailer/Forces/Tires/TireRR ==
  note: Insert your tire model here.
  Sync_In : Inport  OutDataType=sfix(16)  OutScaling=2^0
  Load : Inport  Port=2  OutDataType=sfix(16)  OutScaling=2^0
  vxtrans : Inport  Port=3  OutDataType=sfix(16)  OutScaling=2^0
  vytrans : Inport  Port=4  OutDataType=sfix(16)  OutScaling=2^0
  Rim_rotv : Inport  Port=5  OutDataType=sfix(16)  OutScaling=2^0
  Rim_turnv : Inport  Port=6  OutDataType=sfix(16)  OutScaling=2^0
  InclinAngle : Inport  Port=7  OutDataType=sfix(16)  OutScaling=2^0
  muRoad : Inport  Port=8  OutDataType=sfix(16)  OutScaling=2^0
  Ground{1..11} (11 alike) : Ground
  Terminator{,1..6,12} (8 alike) : Terminator
  Slp : Outport  OutDataType=sfix(16)  OutScaling=2^0
  Alpha : Outport  Port=2  OutDataType=sfix(16)  OutScaling=2^0
  TurnSlp : Outport  Port=3  OutDataType=sfix(16)  OutScaling=2^0
  rBelt_eff : Outport  Port=4  OutDataType=sfix(16)  OutScaling=2^0
  vBelt : Outport  Port=5  OutDataType=sfix(16)  OutScaling=2^0
  LongFrc : Outport  Port=6  OutDataType=sfix(16)  OutScaling=2^0
  SideFrc : Outport  Port=7  OutDataType=sfix(16)  OutScaling=2^0
  LoadFrc : Outport  Port=8  OutDataType=sfix(16)  OutScaling=2^0
  OverturnTrq : Outport  Port=9  OutDataType=sfix(16)  OutScaling=2^0
  RollResist : Outport  Port=10  OutDataType=sfix(16)  OutScaling=2^0
  AlignTrq : Outport  Port=11  OutDataType=sfix(16)  OutScaling=2^0
  wires:
  Ground11/1 -> vBelt/1
  Ground10/1 -> rBelt_eff/1
  Ground9/1 -> TurnSlp/1
  Rim_turnv/1 -> Terminator6/1
  Sync_In/1 -> Terminator12/1
  Ground2/1 -> Alpha/1
  Ground3/1 -> LongFrc/1
  Ground4/1 -> SideFrc/1
  Ground5/1 -> OverturnTrq/1
  vxtrans/1 -> Terminator1/1
  vytrans/1 -> Terminator2/1
  Rim_rotv/1 -> Terminator3/1
  InclinAngle/1 -> Terminator4/1
  muRoad/1 -> Terminator5/1
  Load/1 -> Terminator/1
  Ground1/1 -> Slp/1
  Ground6/1 -> LoadFrc/1
  Ground7/1 -> RollResist/1
  Ground8/1 -> AlignTrq/1

== system AccelCtrl_ACC/CarMaker/VehicleControl/AccelCtrl/ACC ECU/ACC Control/Desired Distance Calculation with time gap ==
  Target.dv : Inport  OutDataType=sfix(16)  OutScaling=2^0
  desired time gap : Inport  Port=2  OutDataType=sfix(16)  OutScaling=2^0
  Enable : EnablePort
  Add : Sum  OutDataType=sfix(16)  OutScaling=2^-10  SaturateOnIntegerOverflow=on  OutDataTypeStr=Inherit: Same as first input
  MinMax : MinMax  Function=max  Inputs=2  OutDataType=sfix(16)  OutScaling=2^0  SaturateOnIntegerOverflow=on  InputSameDT=on
  Product : Product  OutDataType=sfix(16)  OutScaling=2^0  SaturateOnIntegerOverflow=on  OutDataTypeStr=Inherit: Same as first input
  Read Car.v[m/s] : CarMaker4SL/Read CM Dict  xname=Car.v  xsync=off
  Read init min distance from Inf : CarMaker4SL/Read CM Parameter  xfile=Vehicle  xkey=AccelCtrl.ACC.DistMin  xnout=1  xdefaults=20  xmuxed=off
  Write desired distance : CarMaker4SL/Write CM Dict  xname=AccelCtrl.ACC.DesiredDist  xsync=off
  desired distance : Outport  OutDataType=sfix(16)  OutScaling=2^0  InitialOutput=0
  wires:
  Read init min distance from Inf/1 -> MinMax/2
  MinMax/1 -> Write desired distance/1, desired distance/1
  Target.dv/1 -> Add/1
  desired time gap/1 -> Product/1
  Add/1 -> Product/2
  Product/1 -> MinMax/1
  Read Car.v[m/s]/1 -> Add/2

== system AccelCtrl_ACC/CarMaker/VehicleControl/AccelCtrl/ACC ECU/ACC Control/Distance Control Algorithm ==
  Target.ds[m] : Inport  OutDataType=sfix(16)  OutScaling=2^0
  Target.dv[m/s] : Inport  Port=2  OutDataType=sfix(16)  OutScaling=2^0
  desired distance[m] : Inport  Port=3  OutDataType=sfix(16)  OutScaling=2^0
  ax speed control : Inport  Port=4  OutDataType=sfix(16)  OutScaling=2^0
  -2.5<=ax<=1 : Saturate  UpperLimit=1  LowerLimit=-2.5
  desired ax : Subsystem
  "  limited ax" : Outport  OutDataType=sfix(16)  OutScaling=2^0  InitialOutput=0
  wires:
  desired ax/1(desired ax) -> -2.5<=ax<=1/1
  -2.5<=ax<=1/1 -> "  limited ax"/1
  Target.ds[m]/1 -> desired ax/1(Target.ds[m])
  Target.dv[m/s]/1 -> desired ax/2(Target.dv[m/s])
  desired distance[m]/1 -> desired ax/3(desired distance[m])
  ax speed control/1 -> desired ax/4(ax speed control)

== system AccelCtrl_ACC/CarMaker/VehicleControl/AccelCtrl/ACC ECU/ACC Control/Speed Control Algorithm ==
  desire speed[m/s] : Inport  OutDataType=sfix(16)  OutScaling=2^0
  -0.35<=ax<=1 : Saturate  UpperLimit=1  LowerLimit=-0.35
  desired ax : Subsystem
  ax speed control : Outport  OutDataType=sfix(16)  OutScaling=2^0  InitialOutput=0
  wires:
  -0.35<=ax<=1/1 -> ax speed control/1
  desired ax/1(desired ax) -> -0.35<=ax<=1/1
  desire speed[m/s]/1 -> desired ax/1(desire speed[m/s])

== system AccelCtrl_ACC/CarMaker/VehicleControl/AccelCtrl/ACC ECU/ACC User Input/Init Desired time gap quantity ==
  "Init desired time gap " : Inport  OutDataType=sfix(16)  OutScaling=2^0
  Trigger : TriggerPort
  Write init time gap : CarMaker4SL/Write CM Dict  xname=AccelCtrl.ACC.DesiredTGap  xsync=off
  wires:
  "Init desired time gap "/1 -> Write init time gap/1

== system AccelCtrl_ACC/CarMaker/VehicleControl/AccelCtrl/AccelCtrl/PI-Controller/Integrator ==
  I-Part : Inport  OutDataType=sfix(16)  OutScaling=2^0
  AxCtrl On : Inport  Port=2  OutDataType=sfix(16)  OutScaling=2^0
  Init I-part : Inport  Port=3  OutDataType=sfix(16)  OutScaling=2^0
  Add1 : Sum  OutDataType=sfix(16)  OutScaling=2^-10  SaturateOnIntegerOverflow=on  OutDataTypeStr=Inherit: Same as first input
  Memory : Memory
  Saturation : Saturate  UpperLimit=1  LowerLimit=-1
  Switch Ax  Init I-Part : Switch  Threshold=1  SaturateOnIntegerOverflow=on
  "I-part tot " : Outport  OutDataType=sfix(16)  OutScaling=2^0
  wires:
  Init I-part/1 -> Switch Ax  Init I-Part/3
  Memory/1 -> Switch Ax  Init I-Part/1
  AxCtrl On/1 -> Switch Ax  Init I-Part/2
  I-Part/1 -> Add1/1
  Add1/1 -> "I-part tot "/1, Saturation/1
  Switch Ax  Init I-Part/1 -> Add1/2
  Saturation/1 -> Memory/1

== system AccelCtrl_ACC/CarMaker/VehicleControl/AccelCtrl/ACC ECU/ACC Control/Distance Control Algorithm/desired ax ==
  note: delta_ds
  note: desired ax = (target.ds-desired.distance)/(kd)+target.dv/kv
  Target.ds[m] : Inport  OutDataType=sfix(16)  OutScaling=2^0
  Target.dv[m/s] : Inport  Port=2  OutDataType=sfix(16)  OutScaling=2^0
  desired distance[m] : Inport  Port=3  OutDataType=sfix(16)  OutScaling=2^0
  ax speed control : Inport  Port=4  OutDataType=sfix(16)  OutScaling=2^0
  Add : Sum  OutDataType=sfix(16)  OutScaling=2^-10  SaturateOnIntegerOverflow=on  OutDataTypeStr=Inherit: Same as first input
  Divide : Product  Inputs=*/  OutDataType=sfix(16)  OutScaling=2^-10  SaturateOnIntegerOverflow=on  OutDataTypeStr=Inherit: Same as first input
  Divide1 : Product  Inputs=*/  OutDataType=sfix(16)  OutScaling=2^-10  SaturateOnIntegerOverflow=on  OutDataTypeStr=Inherit: Same as first input
  MinMax : MinMax  Inputs=2  OutDataType=sfix(16)  OutScaling=2^0  SaturateOnIntegerOverflow=on  InputSameDT=on
  Read init distctrl.kd from Inf : CarMaker4SL/Read CM Parameter  xfile=Vehicle  xkey=AccelCtrl.ACC.DistCtrl.kd  xnout=1  xdefaults=36  xmuxed=off
  Read init distctrl.kv from Inf1 : CarMaker4SL/Read CM Parameter  xfile=Vehicle  xkey=AccelCtrl.ACC.DistCtrl.kv  xnout=1  xdefaults=2  xmuxed=off
  Subtract : Sum  Inputs=+-  OutDataType=sfix(16)  OutScaling=2^-10  SaturateOnIntegerOverflow=on  OutDataTypeStr=Inherit: Same as first input
  desired ax : Outport  OutDataType=sfix(16)  OutScaling=2^0
  wires:
  Read init distctrl.kv from Inf1/1 -> Divide1/2
  Read init distctrl.kd from Inf/1 -> Divide/2
  Target.dv[m/s]/1 -> Divide1/1
  Target.ds[m]/1 -> Subtract/1
  desired distance[m]/1 -> Subtract/2
  Subtract/1 -> Divide/1
  Divide/1 -> Add/1
  Divide1/1 -> Add/2
  Add/1 -> MinMax/1
  ax speed control/1 -> MinMax/2
  MinMax/1 -> desired ax/1

== system AccelCtrl_ACC/CarMaker/VehicleControl/AccelCtrl/ACC ECU/ACC Control/Speed Control Algorithm/desired ax ==
  desire speed[m/s] : Inport  OutDataType=sfix(16)  OutScaling=2^0
  Divide : Product  Inputs=*/  OutDataType=sfix(16)  OutScaling=2^-10  SaturateOnIntegerOverflow=on  OutDataTypeStr=Inherit: Same as first input
  Read Car.v[m/s] : CarMaker4SL/Read CM Dict  xname=Car.v  xsync=off
  Read init spdctrl.kv from Inf : CarMaker4SL/Read CM Parameter  xfile=Vehicle  xkey=AccelCtrl.ACC.SpdCtrl.kv  xnout=1  xdefaults=13  xmuxed=off
  Sum : Sum  Inputs=|+-  OutDataType=sfix(16)  OutScaling=2^0  SaturateOnIntegerOverflow=on  OutDataTypeStr=Inherit: Same as first input
  desired ax : Outport  OutDataType=sfix(16)  OutScaling=2^0
  wires:
  Read init spdctrl.kv from Inf/1 -> Divide/2
  Sum/1 -> Divide/1
  Read Car.v[m/s]/1 -> Sum/2
  desire speed[m/s]/1 -> Sum/1
  Divide/1 -> desired ax/1
